simulink model "Simulink_model"  (R2023b)
settings: Solver=VariableStepAuto  StartTime=0.0  StopTime=10  RelTol=1e-3
settings Model: Creator=user  LastModifiedBy=user

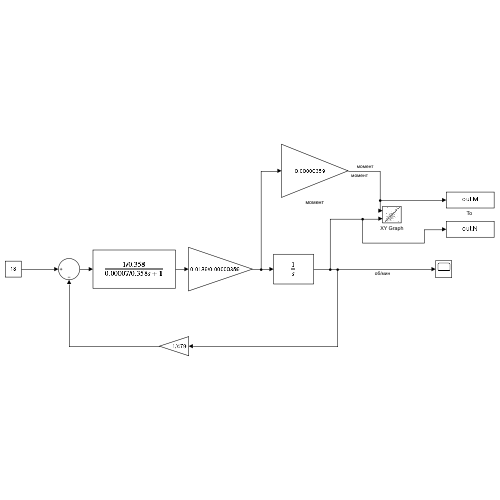
[thumbnail: Simulink's stored preview of the top-level diagram]
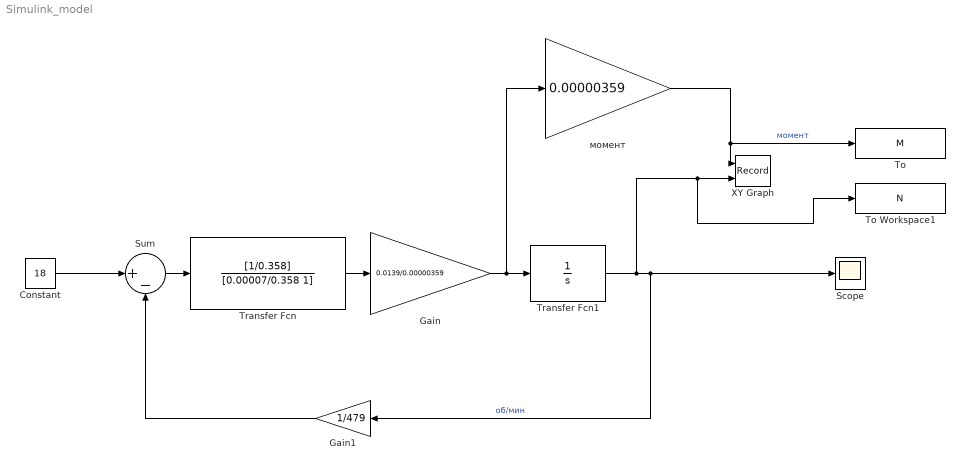
== system Simulink_model ==
  Constant : Constant  Value=18
  Gain : Gain  Gain=0.0139/0.00000359
  Gain1 : Gain  Gain=1/479
  Scope : Scope
  Sum : Sum  Inputs=|+-
  "To " : ToWorkspace  VariableName=M  SaveFormat=Timeseries  SampleTime=-1
  To Workspace1 : ToWorkspace  VariableName=N  SaveFormat=Timeseries  SampleTime=-1
  Transfer Fcn : TransferFcn  Numerator=[1/0.358]  Denominator=[0.00007/0.358 1]
  Transfer Fcn1 : TransferFcn  Denominator=[1 0]
  XY Graph : Record  FileSettingsInternal="{\"entries\":[{\"content\":{\"excelSettings\":{\"content\":{},\"type\":\"Streamout.ExcelSettings\"}},\"type\":\"Streamout.FileSettingStorage\",\"uuid\":\"\"}],\"packageUris\":[\"http:\\/\\/schema.mathworks.com\\/mf0\\/streamout_blocks\\/R2020a\"],\"version\":\"1.0\"}"  Layout=[1 1]  SignalsInternal="{\"entries\":[{\"content\":{\"signals\":[{\"content\":{\"blockPath\":[],\"dimensions\":[1],\"domain\":\"\",\"lineColor\":\"#a2142f\",\"plots\":[1],\"port\":1,\"sid\":[\"\"],\"signalID\":164,\"signalName\":\"момент\"},\"type\":\"RecordBlkView.Signal\",\"uuid\":\"\"},{\"content\":{\"blockPath\":[],\"dimensions\":[1],\"domain\":\"\",\"lineColor\":\"#139fff\",\"plots\":[1],\"port\":2,\"sid\":[\"\"],\"signalID\":168,\"signalName\":\"об\\/мин\"},\"type\":\"RecordBlkView.Signal\",\"uuid\":\"\"}]},\"type\":\"RecordBlkView.InputSignals\",\"uuid\":\"\"}],\"packageUris\":[\"http:\\/\\/schema.mathworks.com\\/mf0\\/streamout_blocks\\/R2020a\"],\"version\":\"1.0\"}"  VisualizationBindings="{\"xyplotplugin\":{\"info\":[{\"series\":[{\"bindingParametersList\":[{\"parameter\":\"X-Axis\",\"signalID\":164,\"signalName\":\"момент\"},{\"parameter\":\"Y-Axis\",\"signalID\":168,\"signalName\":\"об\\/мин\"}],\"seriesID\":50958}],\"subplotID\":1}]}}"  CompatibilityTag=XY
  момент : Gain  Gain=0.00000359
  wires:
  Sum/1 -> Transfer Fcn/1
  Gain/1 -> момент/1, Transfer Fcn1/1
  Transfer Fcn/1 -> Gain/1
  Transfer Fcn1/1 -> To Workspace1/1, XY Graph/2, Gain1/1, Scope/1  "об/мин"
  Constant/1 -> Sum/1
  Gain1/1 -> Sum/2
  момент/1 -> "To "/1, XY Graph/1  "момент"
